simulink model "mmc_classical_complete"  (R2022b)
settings: Solver=VariableStepAuto  StartTime=0.0  StopTime=0.2  RelTol=1e-3
model workspace (MAT data in the model file):
  phase_shift : Simulink.Parameter (value not decoded)
symbols that are objects in the model workspace (value not decoded): phase_shift
undefined symbols (not defined in the file or in its folder): cap_ref, itr, KiC, KpC, Vdc
libraries: spsIGBTDiodeLib x48, spsSeriesRLCBranchLib x33, slpidlib x30, spsVoltageMeasurementLib x27, spsTriangleGeneratorLib x24, spsCurrentMeasurementLib x7, spsDCVoltageSourceLib x1, spspowerguiLib x1
(part 3 of 4)

== system mmc_classical_complete/Phase_2_driver/Capacitor voltage control5 ==
  Add3 : Sum  Inputs=+-
  Constant2 : Constant  Value=cap_ref
  Constant3 : Constant
  Constant4 : Constant  Value=-1
  PID Controller2 : slpidlib/PID Controller  Controller=PID  Form=Parallel  TimeDomain=Continuous-time  UseExternalTs=off  SampleTime=-1  IntegratorMethod=Forward Euler  FilterMethod=Forward Euler  ControllerParametersSource=internal  P=KpC  I=KiC  UseKiTs=off  D=0  N=100  UseFilter=on  TunerSelectOption=Transfer Function Based (PID Tuner App)  InitialConditionSource=internal  InitialConditionForIntegrator=0  InitialConditionForFilter=0  DifferentiatorICPrevScaledInput=0  ExternalReset=none  TrackingMode=off  Kt=1  LimitOutput=off  SatLimitsSource=internal  UpperSaturationLimit=inf  LowerSaturationLimit=-inf  LinearizeAsGain=on  AntiWindupMode=none  Kb=1  LimitIntegrator=off  UpperIntegratorSaturationLimit=inf  LowerIntegratorSaturationLimit=-inf  POutMin=[]  POutMax=[]  IOutMin=[]  IOutMax=[]  DOutMin=[]  DOutMax=[]  NOutMin=[]  NOutMax=[]  SumOutMin=[]  SumOutMax=[]  SaturationOutMin=[]  SaturationOutMax=[]  PParamMin=[]  PParamMax=[]  IParamMin=[]  IParamMax=[]  DParamMin=[]  DParamMax=[]  NParamMin=[]  NParamMax=[]  KbParamMin=[]  KbParamMax=[]  KtParamMin=[]  KtParamMax=[]  KbOutMin=[]  KbOutMax=[]  KtOutMin=[]  KtOutMax=[]  IntegratorOutMin=[]  IntegratorOutMax=[]  FilterOutMin=[]  FilterOutMax=[]  SumI1OutMin=[]  SumI1OutMax=[]  SumI2OutMin=[]  SumI2OutMax=[]  SumI3OutMin=[]  SumI3OutMax=[]  SumI4OutMin=[]  SumI4OutMax=[]  SumDOutMin=[]  SumDOutMax=[]  DifferentiatorOutMin=[]  DifferentiatorOutMax=[]  FilterDiffOutCoefMin=[]  FilterDiffOutCoefMax=[]  ReciprocalOutMin=[]  ReciprocalOutMax=[]  SumDenOutMin=[]  SumDenOutMax=[]  SumNumOutMin=[]  SumNumOutMax=[]  DivideOutMin=[]  DivideOutMax=[]  UdiffTsProdOutMin=[]  UdiffTsProdOutMax=[]  NTsProdOutMin=[]  NTsProdOutMax=[]  UintegralTsProdOutMin=[]  UintegralTsProdOutMax=[]  UngainTsProdOutMin=[]  UngainTsProdOutMax=[]  ClampingZeroOutDataTypeStr=Inherit: Inherit via back propagation  ClampingZeroOutMin=[]  ClampingZeroOutMax=[]  FilterDenConstantOutDataTypeStr=Inherit: Inherit via back propagation  FilterDenConstantOutMin=[]  FilterDenConstantOutMax=[]  PCopyOutDataTypeStr=Inherit: Inherit via back propagation  PCopyOutMin=[]  PCopyOutMax=[]  NCopyOutDataTypeStr=Inherit: Inherit via back propagation  NCopyOutMin=[]  NCopyOutMax=[]  IntegratorContinuousStateAttributes=''  IntegratorStateMustResolveToSignalObject=off  IntegratorRTWStateStorageClass=Auto  FilterContinuousStateAttributes=''  FilterStateMustResolveToSignalObject=off  FilterRTWStateStorageClass=Auto  ParallelPVariant=InternalParameters  IdealPVariant=Disabled  IVariant=InternalParameters  DVariant=InternalParameters  IntegratorVariant=Continuous  SatVariant=Disabled  AWVariant=Passthrough  PCopyVariant=Disabled  TRVariant=Disabled  FdbkBlocksVariant=Forward  IdealPFdbkVariant=Disabled  SatFdbkVariant=Disabled  DerivativeFilterVariant=ContFilter  NVariant=InternalParameters  NCopyVariant=Disabled  FilterICVariant=InternalICsFilter  IntegratorICVariant=InternalICs  ExternalResetVariant=Disabled  TRSumVariant=Passthrough  SumFdbkVariant=Disabled  SumVariant=Sum_PID  TsampFilterVariant=InternalTs  TsampNgainVariant=Passthrough  TsampIntegralVariant=Passthrough  ExternalSaturationOutDataTypeStr=Inherit: Same as second input
  Product : Product
  Scope4 : Scope  NumInputPorts=2
  Switch : Switch  SaturateOnIntegerOverflow=off  InputSameDT=off
  tag scope: CC_6_p2=global
  wires:
  Product/1 -> [CC_6_p2]
  Constant3/1 -> Switch/1
  [Vc6_p2] -> Add3/2
  PID Controller2/1 -> Product/1, Scope4/2
  [I_lower_p2] -> Switch/2
  Switch/1 -> Scope4/1, Product/2
  Constant4/1 -> Switch/3
  Constant2/1 -> Add3/1
  Add3/1 -> PID Controller2/1

== system mmc_classical_complete/Phase_2_driver/Capacitor voltage control6 ==
  Add3 : Sum  Inputs=+-
  Constant2 : Constant  Value=cap_ref
  Constant3 : Constant
  Constant4 : Constant  Value=-1
  PID Controller2 : slpidlib/PID Controller  Controller=PID  Form=Parallel  TimeDomain=Continuous-time  UseExternalTs=off  SampleTime=-1  IntegratorMethod=Forward Euler  FilterMethod=Forward Euler  ControllerParametersSource=internal  P=KpC  I=KiC  UseKiTs=off  D=0  N=100  UseFilter=on  TunerSelectOption=Transfer Function Based (PID Tuner App)  InitialConditionSource=internal  InitialConditionForIntegrator=0  InitialConditionForFilter=0  DifferentiatorICPrevScaledInput=0  ExternalReset=none  TrackingMode=off  Kt=1  LimitOutput=off  SatLimitsSource=internal  UpperSaturationLimit=inf  LowerSaturationLimit=-inf  LinearizeAsGain=on  AntiWindupMode=none  Kb=1  LimitIntegrator=off  UpperIntegratorSaturationLimit=inf  LowerIntegratorSaturationLimit=-inf  POutMin=[]  POutMax=[]  IOutMin=[]  IOutMax=[]  DOutMin=[]  DOutMax=[]  NOutMin=[]  NOutMax=[]  SumOutMin=[]  SumOutMax=[]  SaturationOutMin=[]  SaturationOutMax=[]  PParamMin=[]  PParamMax=[]  IParamMin=[]  IParamMax=[]  DParamMin=[]  DParamMax=[]  NParamMin=[]  NParamMax=[]  KbParamMin=[]  KbParamMax=[]  KtParamMin=[]  KtParamMax=[]  KbOutMin=[]  KbOutMax=[]  KtOutMin=[]  KtOutMax=[]  IntegratorOutMin=[]  IntegratorOutMax=[]  FilterOutMin=[]  FilterOutMax=[]  SumI1OutMin=[]  SumI1OutMax=[]  SumI2OutMin=[]  SumI2OutMax=[]  SumI3OutMin=[]  SumI3OutMax=[]  SumI4OutMin=[]  SumI4OutMax=[]  SumDOutMin=[]  SumDOutMax=[]  DifferentiatorOutMin=[]  DifferentiatorOutMax=[]  FilterDiffOutCoefMin=[]  FilterDiffOutCoefMax=[]  ReciprocalOutMin=[]  ReciprocalOutMax=[]  SumDenOutMin=[]  SumDenOutMax=[]  SumNumOutMin=[]  SumNumOutMax=[]  DivideOutMin=[]  DivideOutMax=[]  UdiffTsProdOutMin=[]  UdiffTsProdOutMax=[]  NTsProdOutMin=[]  NTsProdOutMax=[]  UintegralTsProdOutMin=[]  UintegralTsProdOutMax=[]  UngainTsProdOutMin=[]  UngainTsProdOutMax=[]  ClampingZeroOutDataTypeStr=Inherit: Inherit via back propagation  ClampingZeroOutMin=[]  ClampingZeroOutMax=[]  FilterDenConstantOutDataTypeStr=Inherit: Inherit via back propagation  FilterDenConstantOutMin=[]  FilterDenConstantOutMax=[]  PCopyOutDataTypeStr=Inherit: Inherit via back propagation  PCopyOutMin=[]  PCopyOutMax=[]  NCopyOutDataTypeStr=Inherit: Inherit via back propagation  NCopyOutMin=[]  NCopyOutMax=[]  IntegratorContinuousStateAttributes=''  IntegratorStateMustResolveToSignalObject=off  IntegratorRTWStateStorageClass=Auto  FilterContinuousStateAttributes=''  FilterStateMustResolveToSignalObject=off  FilterRTWStateStorageClass=Auto  ParallelPVariant=InternalParameters  IdealPVariant=Disabled  IVariant=InternalParameters  DVariant=InternalParameters  IntegratorVariant=Continuous  SatVariant=Disabled  AWVariant=Passthrough  PCopyVariant=Disabled  TRVariant=Disabled  FdbkBlocksVariant=Forward  IdealPFdbkVariant=Disabled  SatFdbkVariant=Disabled  DerivativeFilterVariant=ContFilter  NVariant=InternalParameters  NCopyVariant=Disabled  FilterICVariant=InternalICsFilter  IntegratorICVariant=InternalICs  ExternalResetVariant=Disabled  TRSumVariant=Passthrough  SumFdbkVariant=Disabled  SumVariant=Sum_PID  TsampFilterVariant=InternalTs  TsampNgainVariant=Passthrough  TsampIntegralVariant=Passthrough  ExternalSaturationOutDataTypeStr=Inherit: Same as second input
  Product : Product
  Scope4 : Scope  NumInputPorts=2
  Switch : Switch  SaturateOnIntegerOverflow=off  InputSameDT=off
  tag scope: CC_7_p2=global
  wires:
  Add3/1 -> PID Controller2/1
  Constant2/1 -> Add3/1
  Constant4/1 -> Switch/3
  Switch/1 -> Product/2, Scope4/1
  [I_lower_p2] -> Switch/2
  PID Controller2/1 -> Scope4/2, Product/1
  [Vc7_p2] -> Add3/2
  Constant3/1 -> Switch/1
  Product/1 -> [CC_7_p2]

== system mmc_classical_complete/Phase_2_driver/Capacitor voltage control7 ==
  Add3 : Sum  Inputs=+-
  Constant2 : Constant  Value=cap_ref
  Constant3 : Constant
  Constant4 : Constant  Value=-1
  PID Controller2 : slpidlib/PID Controller  Controller=PID  Form=Parallel  TimeDomain=Continuous-time  UseExternalTs=off  SampleTime=-1  IntegratorMethod=Forward Euler  FilterMethod=Forward Euler  ControllerParametersSource=internal  P=KpC  I=KiC  UseKiTs=off  D=0  N=100  UseFilter=on  TunerSelectOption=Transfer Function Based (PID Tuner App)  InitialConditionSource=internal  InitialConditionForIntegrator=0  InitialConditionForFilter=0  DifferentiatorICPrevScaledInput=0  ExternalReset=none  TrackingMode=off  Kt=1  LimitOutput=off  SatLimitsSource=internal  UpperSaturationLimit=inf  LowerSaturationLimit=-inf  LinearizeAsGain=on  AntiWindupMode=none  Kb=1  LimitIntegrator=off  UpperIntegratorSaturationLimit=inf  LowerIntegratorSaturationLimit=-inf  POutMin=[]  POutMax=[]  IOutMin=[]  IOutMax=[]  DOutMin=[]  DOutMax=[]  NOutMin=[]  NOutMax=[]  SumOutMin=[]  SumOutMax=[]  SaturationOutMin=[]  SaturationOutMax=[]  PParamMin=[]  PParamMax=[]  IParamMin=[]  IParamMax=[]  DParamMin=[]  DParamMax=[]  NParamMin=[]  NParamMax=[]  KbParamMin=[]  KbParamMax=[]  KtParamMin=[]  KtParamMax=[]  KbOutMin=[]  KbOutMax=[]  KtOutMin=[]  KtOutMax=[]  IntegratorOutMin=[]  IntegratorOutMax=[]  FilterOutMin=[]  FilterOutMax=[]  SumI1OutMin=[]  SumI1OutMax=[]  SumI2OutMin=[]  SumI2OutMax=[]  SumI3OutMin=[]  SumI3OutMax=[]  SumI4OutMin=[]  SumI4OutMax=[]  SumDOutMin=[]  SumDOutMax=[]  DifferentiatorOutMin=[]  DifferentiatorOutMax=[]  FilterDiffOutCoefMin=[]  FilterDiffOutCoefMax=[]  ReciprocalOutMin=[]  ReciprocalOutMax=[]  SumDenOutMin=[]  SumDenOutMax=[]  SumNumOutMin=[]  SumNumOutMax=[]  DivideOutMin=[]  DivideOutMax=[]  UdiffTsProdOutMin=[]  UdiffTsProdOutMax=[]  NTsProdOutMin=[]  NTsProdOutMax=[]  UintegralTsProdOutMin=[]  UintegralTsProdOutMax=[]  UngainTsProdOutMin=[]  UngainTsProdOutMax=[]  ClampingZeroOutDataTypeStr=Inherit: Inherit via back propagation  ClampingZeroOutMin=[]  ClampingZeroOutMax=[]  FilterDenConstantOutDataTypeStr=Inherit: Inherit via back propagation  FilterDenConstantOutMin=[]  FilterDenConstantOutMax=[]  PCopyOutDataTypeStr=Inherit: Inherit via back propagation  PCopyOutMin=[]  PCopyOutMax=[]  NCopyOutDataTypeStr=Inherit: Inherit via back propagation  NCopyOutMin=[]  NCopyOutMax=[]  IntegratorContinuousStateAttributes=''  IntegratorStateMustResolveToSignalObject=off  IntegratorRTWStateStorageClass=Auto  FilterContinuousStateAttributes=''  FilterStateMustResolveToSignalObject=off  FilterRTWStateStorageClass=Auto  ParallelPVariant=InternalParameters  IdealPVariant=Disabled  IVariant=InternalParameters  DVariant=InternalParameters  IntegratorVariant=Continuous  SatVariant=Disabled  AWVariant=Passthrough  PCopyVariant=Disabled  TRVariant=Disabled  FdbkBlocksVariant=Forward  IdealPFdbkVariant=Disabled  SatFdbkVariant=Disabled  DerivativeFilterVariant=ContFilter  NVariant=InternalParameters  NCopyVariant=Disabled  FilterICVariant=InternalICsFilter  IntegratorICVariant=InternalICs  ExternalResetVariant=Disabled  TRSumVariant=Passthrough  SumFdbkVariant=Disabled  SumVariant=Sum_PID  TsampFilterVariant=InternalTs  TsampNgainVariant=Passthrough  TsampIntegralVariant=Passthrough  ExternalSaturationOutDataTypeStr=Inherit: Same as second input
  Product : Product
  Scope4 : Scope  NumInputPorts=2
  Switch : Switch  SaturateOnIntegerOverflow=off  InputSameDT=off
  tag scope: CC_8_p2=global
  wires:
  Product/1 -> [CC_8_p2]
  Constant3/1 -> Switch/1
  [Vc8_p2] -> Add3/2
  PID Controller2/1 -> Product/1, Scope4/2
  [I_upper_p2] -> Switch/2
  Switch/1 -> Scope4/1, Product/2
  Constant4/1 -> Switch/3
  Constant2/1 -> Add3/1
  Add3/1 -> PID Controller2/1

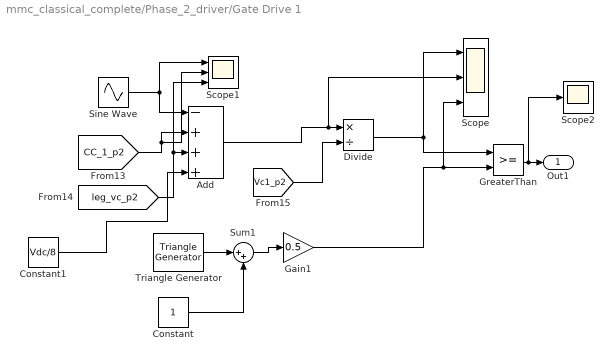
== system mmc_classical_complete/Phase_2_driver/Gate Drive 1 ==
  Add : Sum  Inputs=-+++
  Constant : Constant
  Constant1 : Constant  Value=Vdc/8
  Divide : Product  Inputs=*/
  Gain1 : Gain  Gain=0.5
  GreaterThan : RelationalOperator  OutDataTypeStr=boolean  RndMeth=Simplest  InputSameDT=off
  Scope : Scope  NumInputPorts=3
  Scope1 : Scope  NumInputPorts=3
  Scope2 : Scope
  Sine Wave : Sin  Amplitude=Vdc/8  Frequency=314  Phase=phase_shift  SampleTime=50e-8
  Sum1 : Sum  Inputs=|++
  Triangle Generator : spsTriangleGeneratorLib/Triangle Generator  Freq=tri_freq  Phase=0  Ts=0
  Out1 : Outport
  wires:
  Sum1/1 -> Gain1/1
  Sine Wave/1 -> Scope1/1, Add/1
  [leg_vc_p2] -> Scope1/3, Add/3
  Constant/1 -> Sum1/2
  Add/1 -> Scope/2, Divide/1
  Divide/1 -> GreaterThan/1, Scope/1
  [CC_1_p2] -> Scope1/2, Add/2
  Gain1/1 -> Scope/3, GreaterThan/2
  [Vc1_p2] -> Divide/2
  Triangle Generator/1 -> Sum1/1
  GreaterThan/1 -> Scope2/1, Out1/1
  Constant1/1 -> Add/4

== system mmc_classical_complete/Phase_2_driver/Gate Drive 2 ==
  Add : Sum  Inputs=-+++
  Constant : Constant
  Constant1 : Constant  Value=Vdc/8
  Divide : Product  Inputs=*/
  Gain1 : Gain  Gain=0.5
  GreaterThan : RelationalOperator  OutDataTypeStr=boolean  RndMeth=Simplest  InputSameDT=off
  Sine Wave : Sin  Amplitude=Vdc/8  Frequency=314  Phase=phase_shift  SampleTime=50e-6
  Sum1 : Sum  Inputs=|++
  Triangle Generator : spsTriangleGeneratorLib/Triangle Generator  Freq=tri_freq  Phase=90  Ts=0
  G2 : Outport
  wires:
  GreaterThan/1 -> G2/1
  Triangle Generator/1 -> Sum1/1
  [Vc2_p2] -> Divide/2
  Gain1/1 -> GreaterThan/2
  [CC_2_p2] -> Add/2
  Divide/1 -> GreaterThan/1
  Add/1 -> Divide/1
  Constant/1 -> Sum1/2
  [leg_vc_p2] -> Add/3
  Sine Wave/1 -> Add/1
  Sum1/1 -> Gain1/1
  Constant1/1 -> Add/4

== system mmc_classical_complete/Phase_2_driver/Gate Drive 3 ==
  Add : Sum  Inputs=-+++
  Constant : Constant
  Constant1 : Constant  Value=Vdc/8
  Divide : Product  Inputs=*/
  Gain1 : Gain  Gain=0.5
  GreaterThan : RelationalOperator  OutDataTypeStr=boolean  RndMeth=Simplest  InputSameDT=off
  Sine Wave : Sin  Amplitude=Vdc/8  Frequency=314  Phase=phase_shift  SampleTime=50e-6
  Sum1 : Sum  Inputs=|++
  Triangle Generator : spsTriangleGeneratorLib/Triangle Generator  Freq=tri_freq  Phase=180  Ts=0
  G2 : Outport
  wires:
  Sum1/1 -> Gain1/1
  Sine Wave/1 -> Add/1
  [leg_vc_p2] -> Add/3
  Constant/1 -> Sum1/2
  Add/1 -> Divide/1
  Divide/1 -> GreaterThan/1
  [CC_3_p2] -> Add/2
  Gain1/1 -> GreaterThan/2
  [Vc3_p2] -> Divide/2
  Triangle Generator/1 -> Sum1/1
  GreaterThan/1 -> G2/1
  Constant1/1 -> Add/4

== system mmc_classical_complete/Phase_2_driver/Gate Drive 4 ==
  Add : Sum  Inputs=-+++
  Constant : Constant
  Constant1 : Constant  Value=Vdc/8
  Divide : Product  Inputs=*/
  Gain1 : Gain  Gain=0.5
  GreaterThan : RelationalOperator  OutDataTypeStr=boolean  RndMeth=Simplest  InputSameDT=off
  Sine Wave : Sin  Amplitude=Vdc/8  Frequency=314  Phase=phase_shift  SampleTime=50e-6
  Sum1 : Sum  Inputs=|++
  Triangle Generator : spsTriangleGeneratorLib/Triangle Generator  Freq=tri_freq  Phase=270  Ts=0
  G2 : Outport
  wires:
  GreaterThan/1 -> G2/1
  Triangle Generator/1 -> Sum1/1
  [Vc4_p2] -> Divide/2
  Gain1/1 -> GreaterThan/2
  [CC_4_p2] -> Add/2
  Divide/1 -> GreaterThan/1
  Add/1 -> Divide/1
  Constant/1 -> Sum1/2
  [leg_vc_p2] -> Add/3
  Sine Wave/1 -> Add/1
  Sum1/1 -> Gain1/1
  Constant1/1 -> Add/4

== system mmc_classical_complete/Phase_2_driver/Gate Drive 5 ==
  Add : Sum  Inputs=++++
  Constant : Constant
  Constant1 : Constant  Value=Vdc/8
  Divide : Product  Inputs=*/
  Gain1 : Gain  Gain=0.5
  GreaterThan : RelationalOperator  OutDataTypeStr=boolean  RndMeth=Simplest  InputSameDT=off
  Sine Wave : Sin  Amplitude=Vdc/8  Frequency=314  Phase=phase_shift  SampleTime=50e-6
  Sum1 : Sum  Inputs=|++
  Triangle Generator : spsTriangleGeneratorLib/Triangle Generator  Freq=tri_freq  Phase=0+itr  Ts=0
  G2 : Outport
  wires:
  Sum1/1 -> Gain1/1
  Sine Wave/1 -> Add/1
  [leg_vc_p2] -> Add/3
  Constant/1 -> Sum1/2
  Add/1 -> Divide/1
  Divide/1 -> GreaterThan/1
  [CC_5_p2] -> Add/2
  Gain1/1 -> GreaterThan/2
  [Vc5_p2] -> Divide/2
  Triangle Generator/1 -> Sum1/1
  GreaterThan/1 -> G2/1
  Constant1/1 -> Add/4

== system mmc_classical_complete/Phase_2_driver/Gate Drive 6 ==
  Add : Sum  Inputs=++++
  Constant : Constant
  Constant1 : Constant  Value=Vdc/8
  Divide : Product  Inputs=*/
  Gain1 : Gain  Gain=0.5
  GreaterThan : RelationalOperator  OutDataTypeStr=boolean  RndMeth=Simplest  InputSameDT=off
  Sine Wave : Sin  Amplitude=Vdc/8  Frequency=314  Phase=phase_shift  SampleTime=50e-6
  Sum1 : Sum  Inputs=|++
  Triangle Generator : spsTriangleGeneratorLib/Triangle Generator  Freq=tri_freq  Phase=90+itr  Ts=0
  G2 : Outport
  wires:
  GreaterThan/1 -> G2/1
  Triangle Generator/1 -> Sum1/1
  [Vc6_p2] -> Divide/2
  Gain1/1 -> GreaterThan/2
  [CC_6_p2] -> Add/2
  Divide/1 -> GreaterThan/1
  Add/1 -> Divide/1
  Constant/1 -> Sum1/2
  [leg_vc_p2] -> Add/3
  Sine Wave/1 -> Add/1
  Sum1/1 -> Gain1/1
  Constant1/1 -> Add/4

== system mmc_classical_complete/Phase_2_driver/Gate Drive 7 ==
  Add : Sum  Inputs=++++
  Constant : Constant
  Constant1 : Constant  Value=Vdc/8
  Divide : Product  Inputs=*/
  Gain1 : Gain  Gain=0.5
  GreaterThan : RelationalOperator  OutDataTypeStr=boolean  RndMeth=Simplest  InputSameDT=off
  Sine Wave : Sin  Amplitude=Vdc/8  Frequency=314  Phase=phase_shift  SampleTime=50e-6
  Sum1 : Sum  Inputs=|++
  Triangle Generator : spsTriangleGeneratorLib/Triangle Generator  Freq=tri_freq  Phase=180+itr  Ts=0
  G2 : Outport
  wires:
  Sum1/1 -> Gain1/1
  Sine Wave/1 -> Add/1
  [leg_vc_p2] -> Add/3
  Constant/1 -> Sum1/2
  Add/1 -> Divide/1
  Divide/1 -> GreaterThan/1
  [CC_7_p2] -> Add/2
  Gain1/1 -> GreaterThan/2
  [Vc7_p2] -> Divide/2
  Triangle Generator/1 -> Sum1/1
  GreaterThan/1 -> G2/1
  Constant1/1 -> Add/4

== system mmc_classical_complete/Phase_2_driver/Gate Drive 8 ==
  Add : Sum  Inputs=++++
  Constant : Constant
  Constant1 : Constant  Value=Vdc/8
  Divide : Product  Inputs=*/
  Gain1 : Gain  Gain=0.5
  GreaterThan : RelationalOperator  OutDataTypeStr=boolean  RndMeth=Simplest  InputSameDT=off
  Sine Wave : Sin  Amplitude=Vdc/8  Frequency=314  Phase=phase_shift  SampleTime=50e-6
  Sum1 : Sum  Inputs=|++
  Triangle Generator : spsTriangleGeneratorLib/Triangle Generator  Freq=tri_freq  Phase=270+itr  Ts=0
  G2 : Outport
  wires:
  GreaterThan/1 -> G2/1
  Triangle Generator/1 -> Sum1/1
  [Vc8_p2] -> Divide/2
  Gain1/1 -> GreaterThan/2
  [CC_8_p2] -> Add/2
  Divide/1 -> GreaterThan/1
  Add/1 -> Divide/1
  Constant/1 -> Sum1/2
  [leg_vc_p2] -> Add/3
  Sine Wave/1 -> Add/1
  Sum1/1 -> Gain1/1
  Constant1/1 -> Add/4

== system mmc_classical_complete/Phase_2_driver/Subsystem ==
  G3 : Inport
  IGBT/Diode : spsIGBTDiodeLib/IGBT//Diode  Ron=1e-3  Rs=1e5  Cs=inf  Measurements=on
  IGBT/Diode1 : spsIGBTDiodeLib/IGBT//Diode  Ron=1e-3  Rs=1e5  Cs=inf  Measurements=on
  NOT : Logic  Operator=NOT  IconShape=distinctive  AllPortsSameDT=off  OutDataTypeStr=boolean
  Series RLC Branch : spsSeriesRLCBranchLib/Series RLC Branch  LConnTagsString=__new0  RConnTagsString=__new0  BranchType=C  Resistance=1  Inductance=1e-3  SetiL0=off  InitialCurrent=0  Capacitance=2000e-6  Setx0=on  InitialVoltage=50  Measurements=None
  Voltage Measurement : spsVoltageMeasurementLib/Voltage Measurement  PhasorSimulation=off  OutputType=Complex  PSBequivalent=0
  Input 1 : PMIOPort  Side=Left
  Output 1 : PMIOPort  Port=2  Side=Left
  tag scope: Vc3_p2=global
  wires:
  G3/1 -> IGBT/Diode/1, NOT/1
  NOT/1 -> IGBT/Diode1/1
  Voltage Measurement/1 -> [Vc3_p2]
  connections:
  Voltage Measurement/LConn1 -- IGBT/Diode/LConn1 -- Series RLC Branch/LConn1
  Input 1/RConn1 -- IGBT/Diode1/LConn1 -- IGBT/Diode/RConn1
  Output 1/RConn1 -- IGBT/Diode1/RConn1 -- Voltage Measurement/LConn2 -- Series RLC Branch/RConn1

== system mmc_classical_complete/Phase_2_driver/Subsystem1 ==
  G4 : Inport
  IGBT/Diode : spsIGBTDiodeLib/IGBT//Diode  Ron=1e-3  Rs=1e5  Cs=inf  Measurements=on
  IGBT/Diode1 : spsIGBTDiodeLib/IGBT//Diode  Ron=1e-3  Rs=1e5  Cs=inf  Measurements=on
  NOT : Logic  Operator=NOT  IconShape=distinctive  AllPortsSameDT=off  OutDataTypeStr=boolean
  Series RLC Branch : spsSeriesRLCBranchLib/Series RLC Branch  LConnTagsString=__new0  RConnTagsString=__new0  BranchType=C  Resistance=1  Inductance=1e-3  SetiL0=off  InitialCurrent=0  Capacitance=2000e-6  Setx0=on  InitialVoltage=50  Measurements=None
  Voltage Measurement : spsVoltageMeasurementLib/Voltage Measurement  PhasorSimulation=off  OutputType=Complex  PSBequivalent=0
  Input 2 : PMIOPort  Side=Left
  Output 2 : PMIOPort  Port=2  Side=Left
  tag scope: Vc4_p2=global
  wires:
  Voltage Measurement/1 -> [Vc4_p2]
  NOT/1 -> IGBT/Diode1/1
  G4/1 -> IGBT/Diode/1, NOT/1
  connections:
  Voltage Measurement/LConn2 -- IGBT/Diode1/RConn1 -- Output 2/RConn1 -- Series RLC Branch/RConn1
  Input 2/RConn1 -- IGBT/Diode1/LConn1 -- IGBT/Diode/RConn1
  Voltage Measurement/LConn1 -- IGBT/Diode/LConn1 -- Series RLC Branch/LConn1

== system mmc_classical_complete/Phase_2_driver/Subsystem10 ==
  G7 : Inport
  IGBT/Diode1 : spsIGBTDiodeLib/IGBT//Diode  Ron=1e-3  Rs=1e5  Cs=inf  Measurements=on
  IGBT/Diode2 : spsIGBTDiodeLib/IGBT//Diode  Ron=1e-3  Rs=1e5  Cs=inf  Measurements=on
  NOT : Logic  Operator=NOT  IconShape=distinctive  AllPortsSameDT=off  OutDataTypeStr=boolean
  Series RLC Branch : spsSeriesRLCBranchLib/Series RLC Branch  LConnTagsString=__new0  RConnTagsString=__new0  BranchType=C  Resistance=1  Inductance=1e-3  SetiL0=off  InitialCurrent=0  Capacitance=2000e-6  Setx0=on  InitialVoltage=50  Measurements=None
  Voltage Measurement : spsVoltageMeasurementLib/Voltage Measurement  PhasorSimulation=off  OutputType=Complex  PSBequivalent=0
  Input 3 : PMIOPort  Side=Left
  Output 3 : PMIOPort  Port=2  Side=Left
  tag scope: Vc7_p2=global
  wires:
  Voltage Measurement/1 -> [Vc7_p2]
  NOT/1 -> IGBT/Diode2/1
  G7/1 -> IGBT/Diode1/1, NOT/1
  connections:
  Voltage Measurement/LConn1 -- IGBT/Diode1/LConn1 -- Series RLC Branch/LConn1
  Voltage Measurement/LConn2 -- IGBT/Diode2/RConn1 -- Output 3/RConn1 -- Series RLC Branch/RConn1
  Input 3/RConn1 -- IGBT/Diode2/LConn1 -- IGBT/Diode1/RConn1

== system mmc_classical_complete/Phase_2_driver/Subsystem11 ==
  G6 : Inport
  IGBT/Diode1 : spsIGBTDiodeLib/IGBT//Diode  Ron=1e-3  Rs=1e5  Cs=inf  Measurements=on
  IGBT/Diode2 : spsIGBTDiodeLib/IGBT//Diode  Ron=1e-3  Rs=1e5  Cs=inf  Measurements=on
  NOT : Logic  Operator=NOT  IconShape=distinctive  AllPortsSameDT=off  OutDataTypeStr=boolean
  Series RLC Branch : spsSeriesRLCBranchLib/Series RLC Branch  LConnTagsString=__new0  RConnTagsString=__new0  BranchType=C  Resistance=1  Inductance=1e-3  SetiL0=off  InitialCurrent=0  Capacitance=2000e-6  Setx0=on  InitialVoltage=50  Measurements=None
  Voltage Measurement : spsVoltageMeasurementLib/Voltage Measurement  PhasorSimulation=off  OutputType=Complex  PSBequivalent=0
  Input 4 : PMIOPort  Side=Left
  Output 4 : PMIOPort  Port=2  Side=Left
  tag scope: Vc6_p2=global
  wires:
  G6/1 -> IGBT/Diode1/1, NOT/1
  NOT/1 -> IGBT/Diode2/1
  Voltage Measurement/1 -> [Vc6_p2]
  connections:
  Voltage Measurement/LConn1 -- IGBT/Diode1/LConn1 -- Series RLC Branch/LConn1
  Input 4/RConn1 -- IGBT/Diode2/LConn1 -- IGBT/Diode1/RConn1
  Series RLC Branch/RConn1 -- IGBT/Diode2/RConn1 -- Output 4/RConn1 -- Voltage Measurement/LConn2

== system mmc_classical_complete/Phase_2_driver/Subsystem2 ==
  G5 : Inport
  IGBT/Diode : spsIGBTDiodeLib/IGBT//Diode  Ron=1e-3  Rs=1e5  Cs=inf  Measurements=on
  IGBT/Diode1 : spsIGBTDiodeLib/IGBT//Diode  Ron=1e-3  Rs=1e5  Cs=inf  Measurements=on
  NOT : Logic  Operator=NOT  IconShape=distinctive  AllPortsSameDT=off  OutDataTypeStr=boolean
  Series RLC Branch : spsSeriesRLCBranchLib/Series RLC Branch  LConnTagsString=__new0  RConnTagsString=__new0  BranchType=C  Resistance=1  Inductance=1e-3  SetiL0=off  InitialCurrent=0  Capacitance=2000e-6  Setx0=on  InitialVoltage=50  Measurements=None
  Voltage Measurement : spsVoltageMeasurementLib/Voltage Measurement  PhasorSimulation=off  OutputType=Complex  PSBequivalent=0
  Input 3 : PMIOPort  Side=Left
  Output 3 : PMIOPort  Port=2  Side=Left
  tag scope: Vc5_p2=global
  wires:
  G5/1 -> IGBT/Diode/1, NOT/1
  NOT/1 -> IGBT/Diode1/1
  Voltage Measurement/1 -> [Vc5_p2]
  connections:
  Input 3/RConn1 -- IGBT/Diode1/LConn1 -- IGBT/Diode/RConn1
  Series RLC Branch/RConn1 -- IGBT/Diode1/RConn1 -- Output 3/RConn1 -- Voltage Measurement/LConn2
  Voltage Measurement/LConn1 -- IGBT/Diode/LConn1 -- Series RLC Branch/LConn1

== system mmc_classical_complete/Phase_2_driver/Subsystem3 ==
  G8 : Inport
  IGBT/Diode1 : spsIGBTDiodeLib/IGBT//Diode  Ron=1e-3  Rs=1e5  Cs=inf  Measurements=on
  IGBT/Diode2 : spsIGBTDiodeLib/IGBT//Diode  Ron=1e-3  Rs=1e5  Cs=inf  Measurements=on
  NOT : Logic  Operator=NOT  IconShape=distinctive  AllPortsSameDT=off  OutDataTypeStr=boolean
  Series RLC Branch : spsSeriesRLCBranchLib/Series RLC Branch  LConnTagsString=__new0  RConnTagsString=__new0  BranchType=C  Resistance=1  Inductance=1e-3  SetiL0=off  InitialCurrent=0  Capacitance=2000e-6  Setx0=on  InitialVoltage=50  Measurements=None
  Voltage Measurement : spsVoltageMeasurementLib/Voltage Measurement  PhasorSimulation=off  OutputType=Complex  PSBequivalent=0
  Input 4 : PMIOPort  Side=Left
  Output 4 : PMIOPort  Port=2  Side=Left
  tag scope: Vc8_p2=global
  wires:
  Voltage Measurement/1 -> [Vc8_p2]
  NOT/1 -> IGBT/Diode2/1
  G8/1 -> IGBT/Diode1/1, NOT/1
  connections:
  Voltage Measurement/LConn2 -- IGBT/Diode2/RConn1 -- Output 4/RConn1 -- Series RLC Branch/RConn1
  Input 4/RConn1 -- IGBT/Diode2/LConn1 -- IGBT/Diode1/RConn1
  Voltage Measurement/LConn1 -- IGBT/Diode1/LConn1 -- Series RLC Branch/LConn1

== system mmc_classical_complete/Phase_2_driver/Subsystem6 ==
  G1 : Inport
  IGBT/Diode : spsIGBTDiodeLib/IGBT//Diode  Ron=1e-3  Rs=1e5  Cs=inf  Measurements=on
  IGBT/Diode1 : spsIGBTDiodeLib/IGBT//Diode  Ron=1e-3  Rs=1e5  Cs=inf  Measurements=on
  NOT : Logic  Operator=NOT  IconShape=distinctive  AllPortsSameDT=off  OutDataTypeStr=boolean
  Scope : Scope
  Series RLC Branch : spsSeriesRLCBranchLib/Series RLC Branch  LConnTagsString=__new0  RConnTagsString=__new0  BranchType=C  Resistance=1  Inductance=1e-3  SetiL0=off  InitialCurrent=0  Capacitance=2000e-6  Setx0=on  InitialVoltage=50  Measurements=None
  Voltage Measurement : spsVoltageMeasurementLib/Voltage Measurement  PhasorSimulation=off  OutputType=Complex  PSBequivalent=0
  Input 1 : PMIOPort  Side=Left
  Output 1 : PMIOPort  Port=2  Side=Left
  tag scope: Vc1_p2=global
  wires:
  Voltage Measurement/1 -> [Vc1_p2]
  NOT/1 -> IGBT/Diode1/1, Scope/1
  G1/1 -> IGBT/Diode/1, NOT/1
  connections:
  Series RLC Branch/RConn1 -- Voltage Measurement/LConn2 -- IGBT/Diode1/RConn1 -- Output 1/RConn1
  Input 1/RConn1 -- IGBT/Diode1/LConn1 -- IGBT/Diode/RConn1
  Voltage Measurement/LConn1 -- IGBT/Diode/LConn1 -- Series RLC Branch/LConn1

== system mmc_classical_complete/Phase_2_driver/Subsystem9 ==
  G2 : Inport
  IGBT/Diode : spsIGBTDiodeLib/IGBT//Diode  Ron=1e-3  Rs=1e5  Cs=inf  Measurements=on
  IGBT/Diode1 : spsIGBTDiodeLib/IGBT//Diode  Ron=1e-3  Rs=1e5  Cs=inf  Measurements=on
  NOT : Logic  Operator=NOT  IconShape=distinctive  AllPortsSameDT=off  OutDataTypeStr=boolean
  Series RLC Branch : spsSeriesRLCBranchLib/Series RLC Branch  LConnTagsString=__new0  RConnTagsString=__new0  BranchType=C  Resistance=1  Inductance=1e-3  SetiL0=off  InitialCurrent=0  Capacitance=2000e-6  Setx0=on  InitialVoltage=50  Measurements=None
  Voltage Measurement : spsVoltageMeasurementLib/Voltage Measurement  PhasorSimulation=off  OutputType=Complex  PSBequivalent=0
  Input 1 : PMIOPort  Side=Left
  Output 1 : PMIOPort  Port=2  Side=Left
  tag scope: Vc2_p2=global
  wires:
  Voltage Measurement/1 -> [Vc2_p2]
  NOT/1 -> IGBT/Diode1/1
  G2/1 -> IGBT/Diode/1, NOT/1
  connections:
  Series RLC Branch/RConn1 -- Voltage Measurement/LConn2 -- IGBT/Diode1/RConn1 -- Output 1/RConn1
  Input 1/RConn1 -- IGBT/Diode1/LConn1 -- IGBT/Diode/RConn1
  Voltage Measurement/LConn1 -- IGBT/Diode/LConn1 -- Series RLC Branch/LConn1

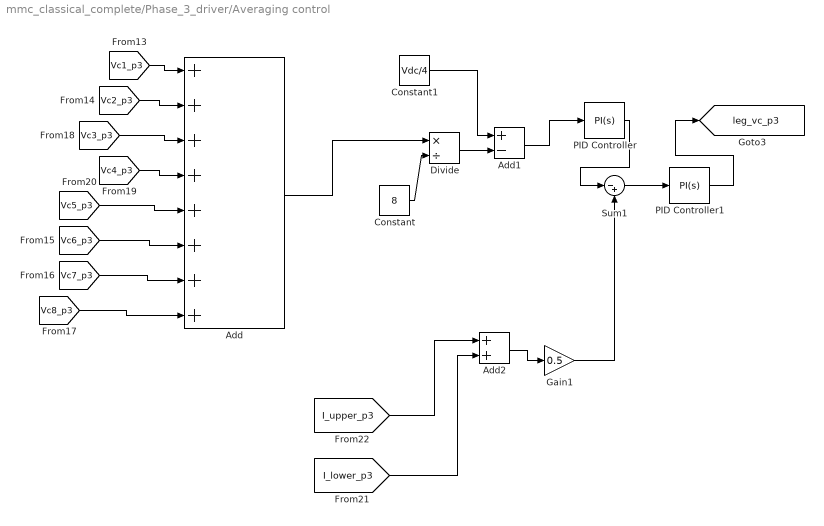
== system mmc_classical_complete/Phase_3_driver/Averaging control  ==
  Add : Sum  Inputs=++++++++
  Add1 : Sum  Inputs=+-
  Add2 : Sum
  Constant : Constant  Value=8
  Constant1 : Constant  Value=Vdc/4
  Divide : Product  Inputs=*/
  Gain1 : Gain  Gain=0.5
  PID Controller : slpidlib/PID Controller  Controller=PI  Form=Parallel  TimeDomain=Continuous-time  UseExternalTs=off  SampleTime=-1  IntegratorMethod=Forward Euler  FilterMethod=Forward Euler  ControllerParametersSource=internal  P=2  I=120  UseKiTs=off  D=0  N=100  UseFilter=on  TunerSelectOption=Transfer Function Based (PID Tuner App)  InitialConditionSource=internal  InitialConditionForIntegrator=0  InitialConditionForFilter=0  DifferentiatorICPrevScaledInput=0  ExternalReset=none  TrackingMode=off  Kt=1  LimitOutput=off  SatLimitsSource=internal  UpperSaturationLimit=inf  LowerSaturationLimit=-inf  LinearizeAsGain=on  AntiWindupMode=none  Kb=1  LimitIntegrator=off  UpperIntegratorSaturationLimit=inf  LowerIntegratorSaturationLimit=-inf  POutMin=[]  POutMax=[]  IOutMin=[]  IOutMax=[]  DOutMin=[]  DOutMax=[]  NOutMin=[]  NOutMax=[]  SumOutMin=[]  SumOutMax=[]  SaturationOutMin=[]  SaturationOutMax=[]  PParamMin=[]  PParamMax=[]  IParamMin=[]  IParamMax=[]  DParamMin=[]  DParamMax=[]  NParamMin=[]  NParamMax=[]  KbParamMin=[]  KbParamMax=[]  KtParamMin=[]  KtParamMax=[]  KbOutMin=[]  KbOutMax=[]  KtOutMin=[]  KtOutMax=[]  IntegratorOutMin=[]  IntegratorOutMax=[]  FilterOutMin=[]  FilterOutMax=[]  SumI1OutMin=[]  SumI1OutMax=[]  SumI2OutMin=[]  SumI2OutMax=[]  SumI3OutMin=[]  SumI3OutMax=[]  SumI4OutMin=[]  SumI4OutMax=[]  SumDOutMin=[]  SumDOutMax=[]  DifferentiatorOutMin=[]  DifferentiatorOutMax=[]  FilterDiffOutCoefMin=[]  FilterDiffOutCoefMax=[]  ReciprocalOutMin=[]  ReciprocalOutMax=[]  SumDenOutMin=[]  SumDenOutMax=[]  SumNumOutMin=[]  SumNumOutMax=[]  DivideOutMin=[]  DivideOutMax=[]  UdiffTsProdOutMin=[]  UdiffTsProdOutMax=[]  NTsProdOutMin=[]  NTsProdOutMax=[]  UintegralTsProdOutMin=[]  UintegralTsProdOutMax=[]  UngainTsProdOutMin=[]  UngainTsProdOutMax=[]  ClampingZeroOutDataTypeStr=Inherit: Inherit via back propagation  ClampingZeroOutMin=[]  ClampingZeroOutMax=[]  FilterDenConstantOutDataTypeStr=Inherit: Inherit via back propagation  FilterDenConstantOutMin=[]  FilterDenConstantOutMax=[]  PCopyOutDataTypeStr=Inherit: Inherit via back propagation  PCopyOutMin=[]  PCopyOutMax=[]  NCopyOutDataTypeStr=Inherit: Inherit via back propagation  NCopyOutMin=[]  NCopyOutMax=[]  IntegratorContinuousStateAttributes=''  IntegratorStateMustResolveToSignalObject=off  IntegratorRTWStateStorageClass=Auto  FilterContinuousStateAttributes=''  FilterStateMustResolveToSignalObject=off  FilterRTWStateStorageClass=Auto  ParallelPVariant=InternalParameters  IdealPVariant=Disabled  IVariant=InternalParameters  DVariant=Disabled  IntegratorVariant=Continuous  SatVariant=Disabled  AWVariant=Passthrough  PCopyVariant=Disabled  TRVariant=Disabled  FdbkBlocksVariant=Forward  IdealPFdbkVariant=Disabled  SatFdbkVariant=Disabled  DerivativeFilterVariant=Disabled  NVariant=Disabled  NCopyVariant=Disabled_SignalSpec  FilterICVariant=Disabled  IntegratorICVariant=InternalICs  ExternalResetVariant=Disabled  TRSumVariant=Passthrough  SumFdbkVariant=Disabled  SumVariant=Sum_PI  TsampFilterVariant=InternalTs  TsampNgainVariant=Passthrough  TsampIntegralVariant=Passthrough  ExternalSaturationOutDataTypeStr=Inherit: Same as second input
  PID Controller1 : slpidlib/PID Controller  Controller=PI  Form=Parallel  TimeDomain=Continuous-time  UseExternalTs=off  SampleTime=-1  IntegratorMethod=Forward Euler  FilterMethod=Forward Euler  ControllerParametersSource=internal  P=1.8  I=100  UseKiTs=off  D=0  N=100  UseFilter=on  TunerSelectOption=Transfer Function Based (PID Tuner App)  InitialConditionSource=internal  InitialConditionForIntegrator=0  InitialConditionForFilter=0  DifferentiatorICPrevScaledInput=0  ExternalReset=none  TrackingMode=off  Kt=1  LimitOutput=off  SatLimitsSource=internal  UpperSaturationLimit=inf  LowerSaturationLimit=-inf  LinearizeAsGain=on  AntiWindupMode=none  Kb=1  LimitIntegrator=off  UpperIntegratorSaturationLimit=inf  LowerIntegratorSaturationLimit=-inf  POutMin=[]  POutMax=[]  IOutMin=[]  IOutMax=[]  DOutMin=[]  DOutMax=[]  NOutMin=[]  NOutMax=[]  SumOutMin=[]  SumOutMax=[]  SaturationOutMin=[]  SaturationOutMax=[]  PParamMin=[]  PParamMax=[]  IParamMin=[]  IParamMax=[]  DParamMin=[]  DParamMax=[]  NParamMin=[]  NParamMax=[]  KbParamMin=[]  KbParamMax=[]  KtParamMin=[]  KtParamMax=[]  KbOutMin=[]  KbOutMax=[]  KtOutMin=[]  KtOutMax=[]  IntegratorOutMin=[]  IntegratorOutMax=[]  FilterOutMin=[]  FilterOutMax=[]  SumI1OutMin=[]  SumI1OutMax=[]  SumI2OutMin=[]  SumI2OutMax=[]  SumI3OutMin=[]  SumI3OutMax=[]  SumI4OutMin=[]  SumI4OutMax=[]  SumDOutMin=[]  SumDOutMax=[]  DifferentiatorOutMin=[]  DifferentiatorOutMax=[]  FilterDiffOutCoefMin=[]  FilterDiffOutCoefMax=[]  ReciprocalOutMin=[]  ReciprocalOutMax=[]  SumDenOutMin=[]  SumDenOutMax=[]  SumNumOutMin=[]  SumNumOutMax=[]  DivideOutMin=[]  DivideOutMax=[]  UdiffTsProdOutMin=[]  UdiffTsProdOutMax=[]  NTsProdOutMin=[]  NTsProdOutMax=[]  UintegralTsProdOutMin=[]  UintegralTsProdOutMax=[]  UngainTsProdOutMin=[]  UngainTsProdOutMax=[]  ClampingZeroOutDataTypeStr=Inherit: Inherit via back propagation  ClampingZeroOutMin=[]  ClampingZeroOutMax=[]  FilterDenConstantOutDataTypeStr=Inherit: Inherit via back propagation  FilterDenConstantOutMin=[]  FilterDenConstantOutMax=[]  PCopyOutDataTypeStr=Inherit: Inherit via back propagation  PCopyOutMin=[]  PCopyOutMax=[]  NCopyOutDataTypeStr=Inherit: Inherit via back propagation  NCopyOutMin=[]  NCopyOutMax=[]  IntegratorContinuousStateAttributes=''  IntegratorStateMustResolveToSignalObject=off  IntegratorRTWStateStorageClass=Auto  FilterContinuousStateAttributes=''  FilterStateMustResolveToSignalObject=off  FilterRTWStateStorageClass=Auto  ParallelPVariant=InternalParameters  IdealPVariant=Disabled  IVariant=InternalParameters  DVariant=Disabled  IntegratorVariant=Continuous  SatVariant=Disabled  AWVariant=Passthrough  PCopyVariant=Disabled  TRVariant=Disabled  FdbkBlocksVariant=Forward  IdealPFdbkVariant=Disabled  SatFdbkVariant=Disabled  DerivativeFilterVariant=Disabled  NVariant=Disabled  NCopyVariant=Disabled_SignalSpec  FilterICVariant=Disabled  IntegratorICVariant=InternalICs  ExternalResetVariant=Disabled  TRSumVariant=Passthrough  SumFdbkVariant=Disabled  SumVariant=Sum_PI  TsampFilterVariant=InternalTs  TsampNgainVariant=Passthrough  TsampIntegralVariant=Passthrough  ExternalSaturationOutDataTypeStr=Inherit: Same as second input
  Sum1 : Sum  Inputs=|-+
  tag scope: leg_vc_p3=global
  wires:
  Gain1/1 -> Sum1/2
  Add/1 -> Divide/1
  Sum1/1 -> PID Controller1/1
  [Vc4_p3] -> Add/4
  PID Controller1/1 -> [leg_vc_p3]
  PID Controller/1 -> Sum1/1
  [I_lower_p3] -> Add2/2
  [Vc8_p3] -> Add/8
  Constant1/1 -> Add1/1
  [Vc7_p3] -> Add/7
  Add1/1 -> PID Controller/1
  [Vc3_p3] -> Add/3
  [Vc5_p3] -> Add/5
  Constant/1 -> Divide/2
  [I_upper_p3] -> Add2/1
  Add2/1 -> Gain1/1
  Divide/1 -> Add1/2
  [Vc2_p3] -> Add/2
  [Vc6_p3] -> Add/6
  [Vc1_p3] -> Add/1

== system mmc_classical_complete/Phase_3_driver/Capacitor voltage control ==
  Add3 : Sum  Inputs=+-
  Constant2 : Constant  Value=cap_ref
  Constant3 : Constant
  Constant4 : Constant  Value=-1
  PID Controller2 : slpidlib/PID Controller  Controller=PI  Form=Parallel  TimeDomain=Continuous-time  UseExternalTs=off  SampleTime=-1  IntegratorMethod=Forward Euler  FilterMethod=Forward Euler  ControllerParametersSource=internal  P=KpC  I=KiC  UseKiTs=off  D=0  N=100  UseFilter=on  TunerSelectOption=Transfer Function Based (PID Tuner App)  InitialConditionSource=internal  InitialConditionForIntegrator=0  InitialConditionForFilter=0  DifferentiatorICPrevScaledInput=0  ExternalReset=none  TrackingMode=off  Kt=1  LimitOutput=off  SatLimitsSource=internal  UpperSaturationLimit=inf  LowerSaturationLimit=-inf  LinearizeAsGain=on  AntiWindupMode=none  Kb=1  LimitIntegrator=off  UpperIntegratorSaturationLimit=inf  LowerIntegratorSaturationLimit=-inf  POutMin=[]  POutMax=[]  IOutMin=[]  IOutMax=[]  DOutMin=[]  DOutMax=[]  NOutMin=[]  NOutMax=[]  SumOutMin=[]  SumOutMax=[]  SaturationOutMin=[]  SaturationOutMax=[]  PParamMin=[]  PParamMax=[]  IParamMin=[]  IParamMax=[]  DParamMin=[]  DParamMax=[]  NParamMin=[]  NParamMax=[]  KbParamMin=[]  KbParamMax=[]  KtParamMin=[]  KtParamMax=[]  KbOutMin=[]  KbOutMax=[]  KtOutMin=[]  KtOutMax=[]  IntegratorOutMin=[]  IntegratorOutMax=[]  FilterOutMin=[]  FilterOutMax=[]  SumI1OutMin=[]  SumI1OutMax=[]  SumI2OutMin=[]  SumI2OutMax=[]  SumI3OutMin=[]  SumI3OutMax=[]  SumI4OutMin=[]  SumI4OutMax=[]  SumDOutMin=[]  SumDOutMax=[]  DifferentiatorOutMin=[]  DifferentiatorOutMax=[]  FilterDiffOutCoefMin=[]  FilterDiffOutCoefMax=[]  ReciprocalOutMin=[]  ReciprocalOutMax=[]  SumDenOutMin=[]  SumDenOutMax=[]  SumNumOutMin=[]  SumNumOutMax=[]  DivideOutMin=[]  DivideOutMax=[]  UdiffTsProdOutMin=[]  UdiffTsProdOutMax=[]  NTsProdOutMin=[]  NTsProdOutMax=[]  UintegralTsProdOutMin=[]  UintegralTsProdOutMax=[]  UngainTsProdOutMin=[]  UngainTsProdOutMax=[]  ClampingZeroOutDataTypeStr=Inherit: Inherit via back propagation  ClampingZeroOutMin=[]  ClampingZeroOutMax=[]  FilterDenConstantOutDataTypeStr=Inherit: Inherit via back propagation  FilterDenConstantOutMin=[]  FilterDenConstantOutMax=[]  PCopyOutDataTypeStr=Inherit: Inherit via back propagation  PCopyOutMin=[]  PCopyOutMax=[]  NCopyOutDataTypeStr=Inherit: Inherit via back propagation  NCopyOutMin=[]  NCopyOutMax=[]  IntegratorContinuousStateAttributes=''  IntegratorStateMustResolveToSignalObject=off  IntegratorRTWStateStorageClass=Auto  FilterContinuousStateAttributes=''  FilterStateMustResolveToSignalObject=off  FilterRTWStateStorageClass=Auto  ParallelPVariant=InternalParameters  IdealPVariant=Disabled  IVariant=InternalParameters  DVariant=Disabled  IntegratorVariant=Continuous  SatVariant=Disabled  AWVariant=Passthrough  PCopyVariant=Disabled  TRVariant=Disabled  FdbkBlocksVariant=Forward  IdealPFdbkVariant=Disabled  SatFdbkVariant=Disabled  DerivativeFilterVariant=Disabled  NVariant=Disabled  NCopyVariant=Disabled_SignalSpec  FilterICVariant=Disabled  IntegratorICVariant=InternalICs  ExternalResetVariant=Disabled  TRSumVariant=Passthrough  SumFdbkVariant=Disabled  SumVariant=Sum_PI  TsampFilterVariant=InternalTs  TsampNgainVariant=Passthrough  TsampIntegralVariant=Passthrough  ExternalSaturationOutDataTypeStr=Inherit: Same as second input
  Product : Product
  Scope4 : Scope  NumInputPorts=2
  Switch : Switch  SaturateOnIntegerOverflow=off  InputSameDT=off
  tag scope: CC_1_p3=global
  wires:
  Product/1 -> [CC_1_p3]
  Constant3/1 -> Switch/1
  [Vc1_p3] -> Add3/2
  PID Controller2/1 -> Product/1, Scope4/2
  [I_upper_p3] -> Switch/2
  Switch/1 -> Scope4/1, Product/2
  Constant4/1 -> Switch/3
  Constant2/1 -> Add3/1
  Add3/1 -> PID Controller2/1

== system mmc_classical_complete/Phase_3_driver/Capacitor voltage control1 ==
  Add3 : Sum  Inputs=+-
  Constant2 : Constant  Value=cap_ref
  Constant3 : Constant
  Constant4 : Constant  Value=-1
  PID Controller2 : slpidlib/PID Controller  Controller=PID  Form=Parallel  TimeDomain=Continuous-time  UseExternalTs=off  SampleTime=-1  IntegratorMethod=Forward Euler  FilterMethod=Forward Euler  ControllerParametersSource=internal  P=KpC  I=KiC  UseKiTs=off  D=0  N=100  UseFilter=on  TunerSelectOption=Transfer Function Based (PID Tuner App)  InitialConditionSource=internal  InitialConditionForIntegrator=0  InitialConditionForFilter=0  DifferentiatorICPrevScaledInput=0  ExternalReset=none  TrackingMode=off  Kt=1  LimitOutput=off  SatLimitsSource=internal  UpperSaturationLimit=inf  LowerSaturationLimit=-inf  LinearizeAsGain=on  AntiWindupMode=none  Kb=1  LimitIntegrator=off  UpperIntegratorSaturationLimit=inf  LowerIntegratorSaturationLimit=-inf  POutMin=[]  POutMax=[]  IOutMin=[]  IOutMax=[]  DOutMin=[]  DOutMax=[]  NOutMin=[]  NOutMax=[]  SumOutMin=[]  SumOutMax=[]  SaturationOutMin=[]  SaturationOutMax=[]  PParamMin=[]  PParamMax=[]  IParamMin=[]  IParamMax=[]  DParamMin=[]  DParamMax=[]  NParamMin=[]  NParamMax=[]  KbParamMin=[]  KbParamMax=[]  KtParamMin=[]  KtParamMax=[]  KbOutMin=[]  KbOutMax=[]  KtOutMin=[]  KtOutMax=[]  IntegratorOutMin=[]  IntegratorOutMax=[]  FilterOutMin=[]  FilterOutMax=[]  SumI1OutMin=[]  SumI1OutMax=[]  SumI2OutMin=[]  SumI2OutMax=[]  SumI3OutMin=[]  SumI3OutMax=[]  SumI4OutMin=[]  SumI4OutMax=[]  SumDOutMin=[]  SumDOutMax=[]  DifferentiatorOutMin=[]  DifferentiatorOutMax=[]  FilterDiffOutCoefMin=[]  FilterDiffOutCoefMax=[]  ReciprocalOutMin=[]  ReciprocalOutMax=[]  SumDenOutMin=[]  SumDenOutMax=[]  SumNumOutMin=[]  SumNumOutMax=[]  DivideOutMin=[]  DivideOutMax=[]  UdiffTsProdOutMin=[]  UdiffTsProdOutMax=[]  NTsProdOutMin=[]  NTsProdOutMax=[]  UintegralTsProdOutMin=[]  UintegralTsProdOutMax=[]  UngainTsProdOutMin=[]  UngainTsProdOutMax=[]  ClampingZeroOutDataTypeStr=Inherit: Inherit via back propagation  ClampingZeroOutMin=[]  ClampingZeroOutMax=[]  FilterDenConstantOutDataTypeStr=Inherit: Inherit via back propagation  FilterDenConstantOutMin=[]  FilterDenConstantOutMax=[]  PCopyOutDataTypeStr=Inherit: Inherit via back propagation  PCopyOutMin=[]  PCopyOutMax=[]  NCopyOutDataTypeStr=Inherit: Inherit via back propagation  NCopyOutMin=[]  NCopyOutMax=[]  IntegratorContinuousStateAttributes=''  IntegratorStateMustResolveToSignalObject=off  IntegratorRTWStateStorageClass=Auto  FilterContinuousStateAttributes=''  FilterStateMustResolveToSignalObject=off  FilterRTWStateStorageClass=Auto  ParallelPVariant=InternalParameters  IdealPVariant=Disabled  IVariant=InternalParameters  DVariant=InternalParameters  IntegratorVariant=Continuous  SatVariant=Disabled  AWVariant=Passthrough  PCopyVariant=Disabled  TRVariant=Disabled  FdbkBlocksVariant=Forward  IdealPFdbkVariant=Disabled  SatFdbkVariant=Disabled  DerivativeFilterVariant=ContFilter  NVariant=InternalParameters  NCopyVariant=Disabled  FilterICVariant=InternalICsFilter  IntegratorICVariant=InternalICs  ExternalResetVariant=Disabled  TRSumVariant=Passthrough  SumFdbkVariant=Disabled  SumVariant=Sum_PID  TsampFilterVariant=InternalTs  TsampNgainVariant=Passthrough  TsampIntegralVariant=Passthrough  ExternalSaturationOutDataTypeStr=Inherit: Same as second input
  Product : Product
  Scope4 : Scope  NumInputPorts=2
  Switch : Switch  SaturateOnIntegerOverflow=off  InputSameDT=off
  tag scope: CC_2_p3=global
  wires:
  Add3/1 -> PID Controller2/1
  Constant2/1 -> Add3/1
  Constant4/1 -> Switch/3
  Switch/1 -> Product/2, Scope4/1
  [I_upper_p3] -> Switch/2
  PID Controller2/1 -> Scope4/2, Product/1
  [Vc2_p3] -> Add3/2
  Constant3/1 -> Switch/1
  Product/1 -> [CC_2_p3]

== system mmc_classical_complete/Phase_3_driver/Capacitor voltage control2 ==
  Add3 : Sum  Inputs=+-
  Constant2 : Constant  Value=cap_ref
  Constant3 : Constant
  Constant4 : Constant  Value=-1
  PID Controller2 : slpidlib/PID Controller  Controller=PID  Form=Parallel  TimeDomain=Continuous-time  UseExternalTs=off  SampleTime=-1  IntegratorMethod=Forward Euler  FilterMethod=Forward Euler  ControllerParametersSource=internal  P=KpC  I=KiC  UseKiTs=off  D=0  N=100  UseFilter=on  TunerSelectOption=Transfer Function Based (PID Tuner App)  InitialConditionSource=internal  InitialConditionForIntegrator=0  InitialConditionForFilter=0  DifferentiatorICPrevScaledInput=0  ExternalReset=none  TrackingMode=off  Kt=1  LimitOutput=off  SatLimitsSource=internal  UpperSaturationLimit=inf  LowerSaturationLimit=-inf  LinearizeAsGain=on  AntiWindupMode=none  Kb=1  LimitIntegrator=off  UpperIntegratorSaturationLimit=inf  LowerIntegratorSaturationLimit=-inf  POutMin=[]  POutMax=[]  IOutMin=[]  IOutMax=[]  DOutMin=[]  DOutMax=[]  NOutMin=[]  NOutMax=[]  SumOutMin=[]  SumOutMax=[]  SaturationOutMin=[]  SaturationOutMax=[]  PParamMin=[]  PParamMax=[]  IParamMin=[]  IParamMax=[]  DParamMin=[]  DParamMax=[]  NParamMin=[]  NParamMax=[]  KbParamMin=[]  KbParamMax=[]  KtParamMin=[]  KtParamMax=[]  KbOutMin=[]  KbOutMax=[]  KtOutMin=[]  KtOutMax=[]  IntegratorOutMin=[]  IntegratorOutMax=[]  FilterOutMin=[]  FilterOutMax=[]  SumI1OutMin=[]  SumI1OutMax=[]  SumI2OutMin=[]  SumI2OutMax=[]  SumI3OutMin=[]  SumI3OutMax=[]  SumI4OutMin=[]  SumI4OutMax=[]  SumDOutMin=[]  SumDOutMax=[]  DifferentiatorOutMin=[]  DifferentiatorOutMax=[]  FilterDiffOutCoefMin=[]  FilterDiffOutCoefMax=[]  ReciprocalOutMin=[]  ReciprocalOutMax=[]  SumDenOutMin=[]  SumDenOutMax=[]  SumNumOutMin=[]  SumNumOutMax=[]  DivideOutMin=[]  DivideOutMax=[]  UdiffTsProdOutMin=[]  UdiffTsProdOutMax=[]  NTsProdOutMin=[]  NTsProdOutMax=[]  UintegralTsProdOutMin=[]  UintegralTsProdOutMax=[]  UngainTsProdOutMin=[]  UngainTsProdOutMax=[]  ClampingZeroOutDataTypeStr=Inherit: Inherit via back propagation  ClampingZeroOutMin=[]  ClampingZeroOutMax=[]  FilterDenConstantOutDataTypeStr=Inherit: Inherit via back propagation  FilterDenConstantOutMin=[]  FilterDenConstantOutMax=[]  PCopyOutDataTypeStr=Inherit: Inherit via back propagation  PCopyOutMin=[]  PCopyOutMax=[]  NCopyOutDataTypeStr=Inherit: Inherit via back propagation  NCopyOutMin=[]  NCopyOutMax=[]  IntegratorContinuousStateAttributes=''  IntegratorStateMustResolveToSignalObject=off  IntegratorRTWStateStorageClass=Auto  FilterContinuousStateAttributes=''  FilterStateMustResolveToSignalObject=off  FilterRTWStateStorageClass=Auto  ParallelPVariant=InternalParameters  IdealPVariant=Disabled  IVariant=InternalParameters  DVariant=InternalParameters  IntegratorVariant=Continuous  SatVariant=Disabled  AWVariant=Passthrough  PCopyVariant=Disabled  TRVariant=Disabled  FdbkBlocksVariant=Forward  IdealPFdbkVariant=Disabled  SatFdbkVariant=Disabled  DerivativeFilterVariant=ContFilter  NVariant=InternalParameters  NCopyVariant=Disabled  FilterICVariant=InternalICsFilter  IntegratorICVariant=InternalICs  ExternalResetVariant=Disabled  TRSumVariant=Passthrough  SumFdbkVariant=Disabled  SumVariant=Sum_PID  TsampFilterVariant=InternalTs  TsampNgainVariant=Passthrough  TsampIntegralVariant=Passthrough  ExternalSaturationOutDataTypeStr=Inherit: Same as second input
  Product : Product
  Scope4 : Scope  NumInputPorts=2
  Switch : Switch  SaturateOnIntegerOverflow=off  InputSameDT=off
  tag scope: CC_3_p3=global
  wires:
  Product/1 -> [CC_3_p3]
  Constant3/1 -> Switch/1
  [Vc3_p3] -> Add3/2
  PID Controller2/1 -> Product/1, Scope4/2
  [I_upper_p3] -> Switch/2
  Switch/1 -> Scope4/1, Product/2
  Constant4/1 -> Switch/3
  Constant2/1 -> Add3/1
  Add3/1 -> PID Controller2/1
